simulink model "level1_challenge2b"  (R2023b)
settings: Solver=VariableStepAuto  StartTime=0.0  StopTime=600  RelTol=1e-3
settings Model: Creator=evreng  LastModifiedBy=evreng

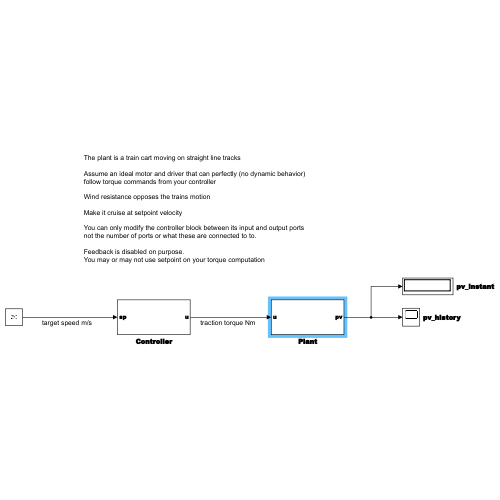
[thumbnail: Simulink's stored preview of the top-level diagram]
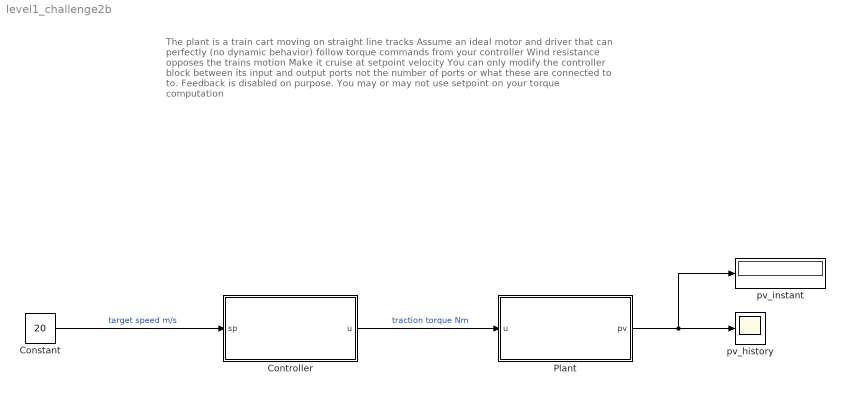
== system level1_challenge2b ==
  note: The plant is a train cart moving on straight line tracks
      |
      | Assume an ideal motor and driver that can perfectly (no dynamic behavior) follow torque commands from your controller
      |
      | Wind resistance opposes the trains motion
      |
      | Make it cruise at setpoint velocity
      |
      | You can only modify the controller block between its input and output ports
      | not the number of ports or what these are connected to to.
      |
      | Feedback is disabled on purpose.
      | You may or may not use setpoint on your torque computation
  Constant : Constant  Value=20
  Controller : Subsystem
  Plant : Subsystem
  pv_history : Scope
  pv_instant : Display
  wires:
  Controller/1(u) -> Plant/1(u)  "traction torque Nm"
  Constant/1 -> Controller/1(sp)  "target speed m/s"
  Plant/1(pv) -> pv_history/1, pv_instant/1

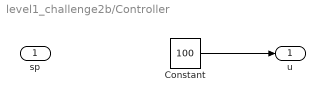
== system level1_challenge2b/Controller ==
  sp : Inport
  Constant : Constant  Value=100
  u : Outport
  wires:
  Constant/1 -> u/1

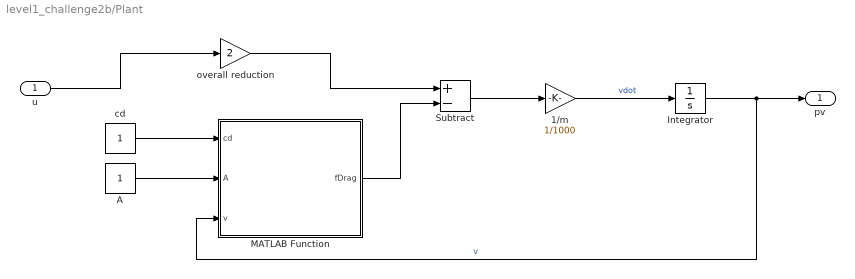
== system level1_challenge2b/Plant ==
  u : Inport
  1/m : Gain  Gain=1/1000
  A : Constant
  Integrator : Integrator
  MATLAB Function : MATLAB Function  TreatAsAtomicUnit=on
  Subtract : Sum  Inputs=+-
  cd : Constant
  overall reduction : Gain  Gain=2
  pv : Outport
  wires:
  u/1 -> overall reduction/1
  1/m/1 -> Integrator/1  "vdot"
  Integrator/1 -> MATLAB Function/3(v), pv/1  "v"
  cd/1 -> MATLAB Function/1(cd)
  A/1 -> MATLAB Function/2(A)
  MATLAB Function/1(fDrag) -> Subtract/2
  Subtract/1 -> 1/m/1
  overall reduction/1 -> Subtract/1

== matlab function level1_challenge2b/Plant/MATLAB Function ==
  data: cd input; fDrag output; A input; v input
function fDrag = airDrag(cd, A, v)
fDrag = 0.5 * cd * A * v ^ 2;
